simulink model "top_model2022b"  (R2022b)
settings: Solver=VariableStepAuto  StartTime=0.0  StopTime=80  FixedStep=0.01  RelTol=1e-3  EnableMultiTasking=on
undefined symbols (not defined in the file): EOL_Vehicle_lf, EOL_Vehicle_lr, EOL_Vehicle_Speed
settings Model: Creator=The MathWorks, Inc.  LastModifiedBy=konur
settings SolverCC: ZeroCrossAlgorithm=Adaptive  AlgebraicLoopSolver=TrustRegion  AutoInsertRateTranBlk=on
settings DataIOCC: LimitDataPoints=on  ReturnWorkspaceOutputs=off
settings OptimizationCC: ReuseModelBlockBuffer=on  LifeSpan=inf
settings DebuggingCC: UnconnectedInputMsg=warning  UnconnectedOutputMsg=warning  UnconnectedLineMsg=warning  AllowSymbolicDim=off  SFUnexpectedBacktrackingDiag=warning  SFNoUnconditionalDefaultTransitionDiag=warning  SFExecutionAtInitializationDiag=none  ArithmeticOperatorsInVariantConditions=warning
settings ModelReferenceCC: EnableRefExpFcnMdlSchedulingChecks=on  PropagateSignalLabelsOutOfModel=off
settings SFSimCC: SimUseLocalCustomCode=off  CustomCodeUndefinedFunction=UseInterfaceOnly
settings RTWCC: RTWUseLocalCustomCode=off
settings CodeAppCC: StateflowObjectComments=on
settings GRTTargetCC: TargetLangStandard=C89/C90 (ANSI)
settings ConfigComp: CovMetricSettings=dw  CovSaveCumulativeToWorkspaceVar=on  CovSaveSingleToWorkspaceVar=on  CovExternalEMLEnable=off

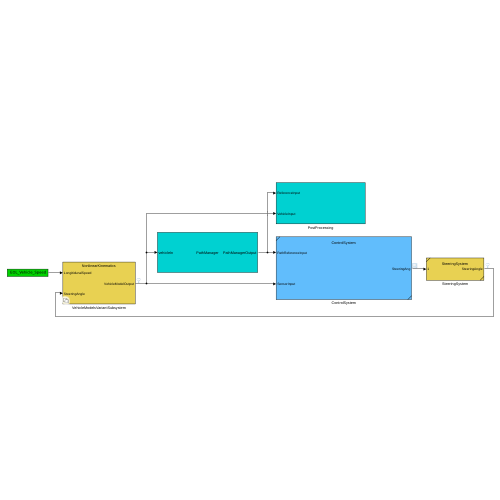
[thumbnail: Simulink's stored preview of the top-level diagram]
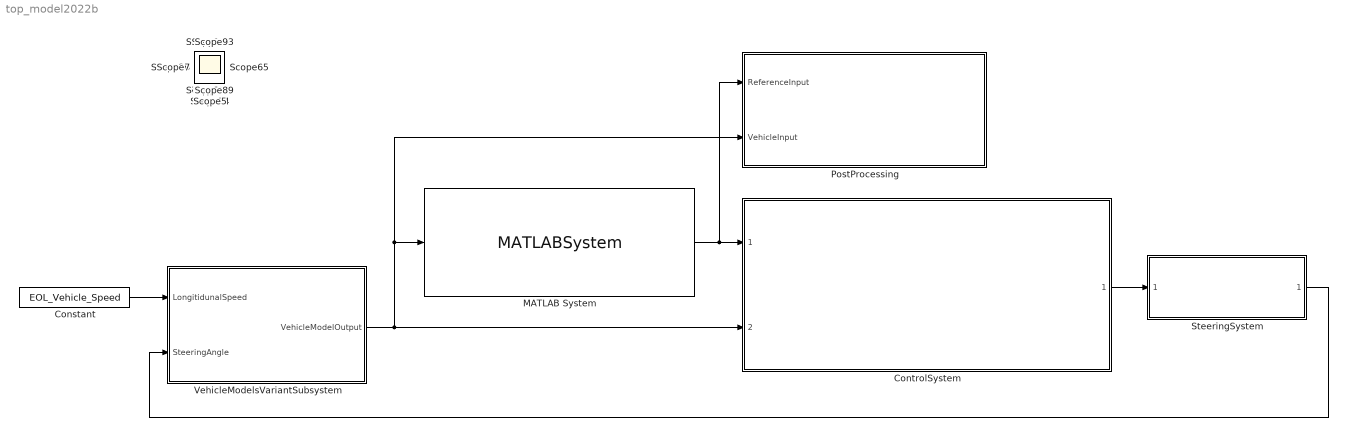
== system top_model2022b ==
  Constant : Constant  Value=EOL_Vehicle_Speed  OutDataTypeStr=double
  ControlSystem : Subsystem  ReferencedSubsystem=ControlSystem
  MATLAB System : MATLABSystem  System=PathManager  SimulateUsing=Interpreted execution
      mask Type: PathManager
      mask Display:
      | disp('PathManager');
      | port_label('input',1,'vehicleIn');
      | port_label('output',1,'PathManagerOutput');
  PostProcessing : Subsystem
  SteeringSystem : Subsystem  ReferencedSubsystem=SteeringSystem
  VehicleModelsVariantSubsystem : Subsystem  Variant=on
  Scope{,1..26} (27 alike) : Scope
  wires:
  ControlSystem/1 -> SteeringSystem/1
  MATLAB System/1 -> PostProcessing/1(ReferenceInput), ControlSystem/1
  VehicleModelsVariantSubsystem/1(VehicleModelOutput) -> MATLAB System/1, PostProcessing/2(VehicleInput), ControlSystem/2
  SteeringSystem/1 -> VehicleModelsVariantSubsystem/2(SteeringAngle)
  Constant/1 -> VehicleModelsVariantSubsystem/1(LongitidunalSpeed)

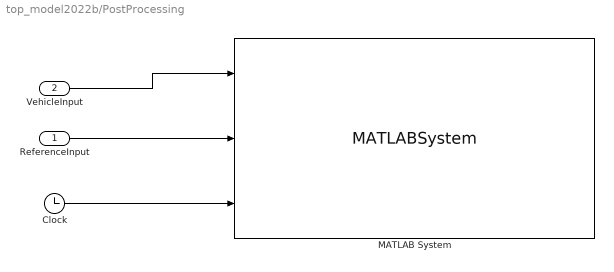
== system top_model2022b/PostProcessing ==
  ReferenceInput : Inport  OutDataTypeStr=Bus: PathManagerOut
  VehicleInput : Inport  Port=2  OutDataTypeStr=Bus: VehicleModelBus
  Clock : Clock
  MATLAB System : MATLABSystem  System=PostProcessing  VehicleBase=EOL_Vehicle_lf + EOL_Vehicle_lr  VehicleFrontAxleToCG=EOL_Vehicle_lf  VehicleRearAxleToCG=EOL_Vehicle_lr  VehicleLength=EOL_Vehicle_lf + EOL_Vehicle_lr + 1.5  VehicleWidth=EOL_Vehicle_Width  InitialPosition_X=EOL_Vehicle_InitX  InitialPosition_Y=EOL_Vehicle_InitY  InitialYawAngle=EOL_Vehicle_INITR  FieldLimitXAxis=[-10 50]  FieldLimitYAxis=[-10 50]  SimulateUsing=Interpreted execution
      mask Type: PostProcessing
      mask Display:
      | disp('PostProcessing');
      | port_label('input',1,'vehicleIn');
      | port_label('input',2,'ReferenceInput');
      | port_label('input',3,'TimeIn');
  wires:
  VehicleInput/1 -> MATLAB System/1
  ReferenceInput/1 -> MATLAB System/2
  Clock/1 -> MATLAB System/3

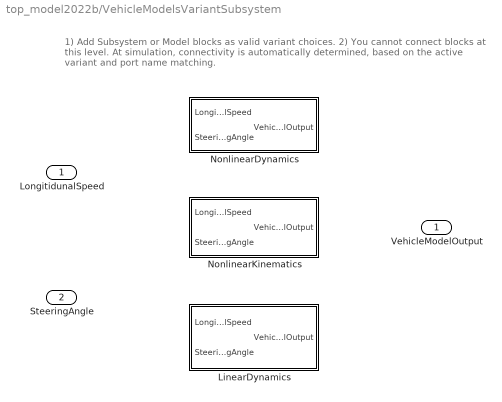
== system top_model2022b/VehicleModelsVariantSubsystem ==
  note: 1) Add Subsystem or Model blocks as valid variant choices.
      | 2) You cannot connect blocks at this level. At simulation, connectivity is automatically
      | determined, based on the active variant and port name matching.
  LongitidunalSpeed : Inport  OutDataTypeStr=double
  SteeringAngle : Inport  Port=2  OutDataTypeStr=double
  LinearDynamics : Subsystem  VariantControl=ModelType==3
  NonlinearDynamics : Subsystem  VariantControl=ModelType==1
  NonlinearKinematics : Subsystem  VariantControl=ModelType==2
  VehicleModelOutput : Outport  OutDataTypeStr=Bus: VehicleModelBus

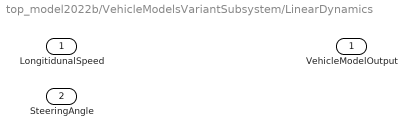
== system top_model2022b/VehicleModelsVariantSubsystem/LinearDynamics ==
  LongitidunalSpeed : Inport
  SteeringAngle : Inport  Port=2
  VehicleModelOutput : Outport  OutDataTypeStr=Bus: VehicleModelBus

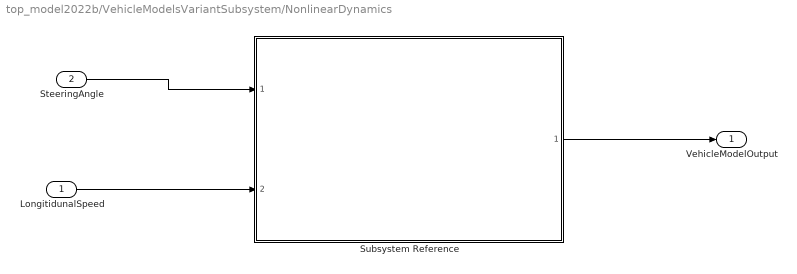
== system top_model2022b/VehicleModelsVariantSubsystem/NonlinearDynamics ==
  LongitidunalSpeed : Inport  OutDataTypeStr=double
  SteeringAngle : Inport  Port=2  OutDataTypeStr=double
  Subsystem Reference : Subsystem  ReferencedSubsystem=VehicleModel
  VehicleModelOutput : Outport  OutDataTypeStr=Bus: VehicleModelBus
  wires:
  LongitidunalSpeed/1 -> Subsystem Reference/2
  SteeringAngle/1 -> Subsystem Reference/1
  Subsystem Reference/1 -> VehicleModelOutput/1

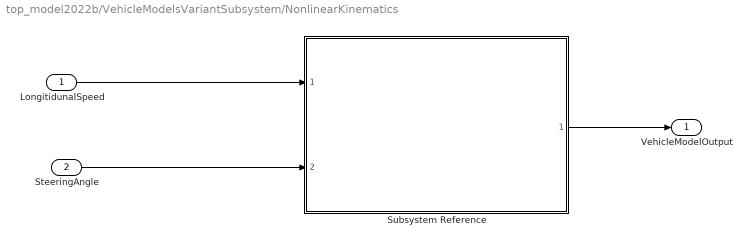
== system top_model2022b/VehicleModelsVariantSubsystem/NonlinearKinematics ==
  LongitidunalSpeed : Inport
  SteeringAngle : Inport  Port=2
  Subsystem Reference : Subsystem  ReferencedSubsystem=KinematicModel
  VehicleModelOutput : Outport  OutDataTypeStr=Bus: VehicleModelBus
  wires:
  LongitidunalSpeed/1 -> Subsystem Reference/1
  SteeringAngle/1 -> Subsystem Reference/2
  Subsystem Reference/1 -> VehicleModelOutput/1
